simulink model "TestMultirotorSimPx4v1_8"  (R2018b)
settings: Solver=VariableStepAuto  StartTime=0.0  StopTime=Simulation.T_END  MaxStep=Simulation.TS_MAX  RelTol=1e-3  EnableMultiTasking=on
PreLoadFcn:
  | % InitializeParameters;
undefined symbols (not defined in the file): Aero, armed, ctrl_state, Initial, Motor, Simulation, Uav, v_att_sp, v_control_mode
libraries: QuaternionLibrary x13, simulink_extras x9, Px4Library x3, dspsigattribs x1, dspstat3 x1, simulink x1
(part 3 of 9)

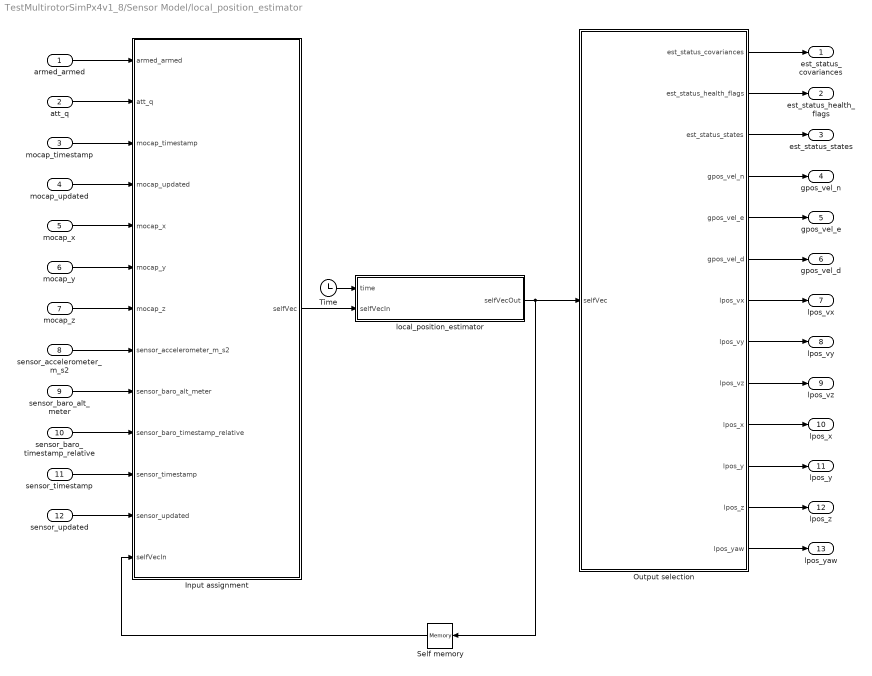
== system TestMultirotorSimPx4v1_8/Sensor Model/local_position_estimator ==
  armed_armed : Inport
  att_q : Inport  Port=2
  mocap_timestamp : Inport  Port=3
  mocap_updated : Inport  Port=4
  mocap_x : Inport  Port=5
  mocap_y : Inport  Port=6
  mocap_z : Inport  Port=7
  sensor_accelerometer_m_s2 : Inport  Port=8
  sensor_baro_alt_meter : Inport  Port=9
  sensor_baro_timestamp_relative : Inport  Port=10
  sensor_timestamp : Inport  Port=11
  sensor_updated : Inport  Port=12
  Input assignment : MATLAB Function  TreatAsAtomicUnit=on
  Output selection : MATLAB Function  TreatAsAtomicUnit=on
  Self memory : Memory  InitialCondition=[0, 0, 0, 0, 0, 0, 0, 0, 0, 0, 0, 0, 0, 0, 0, 0, 0, 0, 0, 0, 0, 0, 0, 0, 0, 0, 0, 0, 0, 0, 0, 0, 0, 0, 0, 0, 0, 0, 0, 0, 0, 0, 0, 0, 0, 0, 0, 0, 0, 0, 0, 0, 0, 0, 0, 0, 0, 0, 0, 0, 0, 0, 0, 0, 0, 0, 0, 0, 0, 0, 0, 0, 0, 0, 0, 0, 0, 0, 0, 0, 0, 0, 0, 0, 0, 0, 0, 0, 0, 0, 0, 0, 0, 0, 0, 0, 0, 0, 0, 0, 0, 0, 0, 0, 0, 0, 0, 0, 0, 0, 0, 0, 0, 0, 0, 0, 0, 0, 0, 0, 0, 0, 0, 0, 0, 0, 0, 0, 0, 0, 0, 8.82050518214, 12.094592431, 13.9876612368, 16.0875642296, 17.8797700658, 19.6465647819, 1e-1, 2.0, 2.0, 2.0, 2^2, 2^0, 2^1, 2^7, 2^1, 2^6, 2^0, 2^4, 2^5, 2^2, 2^3, 0, 10.0, 8, 0, 0, 0, 0, 0, 0, 0, 0, 0, 0, 8, 0, 0, 0, 0, 0, 0, 0, 0, 0, 0, 8, 0, 0, 0, 0, 0, 0, 0, 0, 0, 0, 2*LPE_VXY_PUB*LPE_VXY_PUB, 0, 0, 0, 0, 0, 0, 0, 0, 0, 0, 2*LPE_VXY_PUB*LPE_VXY_PUB, 0, 0, 0, 0, 0, 0, 0, 0, 0, 0, 2*LPE_VXY_PUB*LPE_VXY_PUB, 0, 0, 0, 0, 0, 0, 0, 0, 0, 0, 1e-6, 0, 0, 0, 0, 0, 0, 0, 0, 0, 0, 1e-6, 0, 0, 0, 0, 0, 0, 0, 0, 0, 0, 1e-6, 0, 0, 0, 0, 0, 0, 0, 0, 0, 0, 8, 1.0e6, 0, 0, 0, 0, 0, 0, 0, 0, 0, 0, 0, 0, 0, 0, 0, 0, 0, 0, 0, 0, 0, 0, 0, 0, 0, 0, 0, 0, 0, 0, 0, 0, 0, 0, 0, 0, 0, 0, 0, 0, 0, 0, 0, 0, 0, 0, 0, 0, 0, 0, 0, 0, 0, 0, 0, 0, 0, 0, 0, 0, 0, 0, 0, 0, 0, 0, 0, 0, 0, 0, 0, 0, 0, 0, 0, 0, 0, 0, 0, 0, 0, 0, 0, 0, 0, 0, 0, 0, 0, 0, 0, 0, 0, 0, 0, 0, 0, 0, 0, 0, 0, 0, 0, 0, 0, 0, 0, 0, 0, 0, 0, 0, 0, 0, 0, 0, 0, 0, 2^0, 2^3, 2^1, 2^7, 2^2, 2^6, 2^4, 2^5, 0, LPE_ACC_XY, 0, LPE_ACC_Z, LPE_SAMPLING_PERIOD, LPE_X_LP, 0, 0, 0, 0, 0, 0, LPE_BAR_Z, LPE_SAMPLING_PERIOD, 0, 0, 0, 0, LPE_FAKE_ORIGIN, 0, LPE_FGYRO_HP, LPE_FGYRO_HP, LPE_FLW_QMIN, LPE_FLW_R, LPE_FLW_RR, LPE_FLW_SCALE, LPE_FLW_OFF_Z, LPE_FUSION, 0, LPE_GPS_DELAY, LPE_EPH_MAX, LPE_EPV_MAX, LPE_GPS_VXY, LPE_GPS_VZ, LPE_GPS_XY, LPE_GPS_Z, LPE_LAT, LPE_LON, 0, 0, LPE_LAND_VXY, LPE_LAND_Z, 0, LPE_LDR_OFF_Z, LPE_LDR_Z, 0, 0, 0, 0, 0, 0, 0, LPE_VIC_P, LPE_PN_B, LPE_PN_P, LPE_PN_T, LPE_PN_V, 8, 0, 0, 0, 0, 0, 0, 0, 0, 0, 0, 0, 0, 0, 0, 0, 0, 0, 0, 0, 0, 0, 0, 0, 0, 0, 0, 0, 0, 0, 0, 0, 0, 0, 0, 0, 0, 0, 0, 0, 0, 0, 0, 0, 0, 0, 0, 0, 0, 0, 0, 0, 0, 0, 0, 0, 0, 0, 0, 0, 0, 0, 0, 0, 0, 0, 0, 0, 0, 0, 0, 0, 0, 0, 0, 255, 0, LPE_SNR_OFF_Z, LPE_SNR_Z, 0, 0, 0, 0, 0, 0, 0, 0, 0, 0, 0, 0, 0, 0, 0, 0, 0, 0, 0, 0, 0, 0, 0, 0, 0, 0, 0, 0, 0, 0, 0, 0, 0, 0, 0, 0, 0, 0, 0, 1, 1, LPE_T_MAX_GRADE, 0, 0, 0, 0, 0, 0, 0, 0, 0, 0, 0, LPE_VIS_DELAY, LPE_VIS_XY, LPE_VIS_Z, LPE_VXY_PUB, 0, 0, 0, 0, 0, 0, 0, 0, 0, 0, 0, 0, 0, 0, 0, 0, 0, 0, 0, 0, 0, 0, 0, 0, 0, 0, 0, 0, 0, 0, 0, 0, 0, 0, 0, 0, 0, 0, 0, 0, 0, 0, 0, 0, 0, 0, 0, 0, 0, 0, 0, 0, 0, 0, 0, 0, 0, 0, 0, 0, 0, 0, 0, 0, 0, 0, 0, 0, 0, 0, 0, 0, 0, 0, 0, 0, 0, 0, 0, 0, 0, 0, 0, 0, 0, 0, 0, 0, 0, 0, 0, 0, 0, 0, 0, 0, 0, 0, 0, 0, 0, 0, 0, 0, 0, 0, 0, 0, 0, 0, 1, 1, LPE_SAMPLING_PERIOD, LPE_X_LP, 0, 0, 0, 0, 0, 0, 0, 0, 0, 0, LPE_Z_PUB]
  Time : Clock
  local_position_estimator : MATLAB Function  TreatAsAtomicUnit=on  SystemSampleTime=LPE_SAMPLING_PERIOD
  est_status_covariances : Outport
  est_status_health_flags : Outport  Port=2
  est_status_states : Outport  Port=3
  gpos_vel_n : Outport  Port=4
  gpos_vel_e : Outport  Port=5
  gpos_vel_d : Outport  Port=6
  lpos_vx : Outport  Port=7
  lpos_vy : Outport  Port=8
  lpos_vz : Outport  Port=9
  lpos_x : Outport  Port=10
  lpos_y : Outport  Port=11
  lpos_z : Outport  Port=12
  lpos_yaw : Outport  Port=13
  wires:
  Output selection/13(lpos_yaw) -> lpos_yaw/1
  Output selection/12(lpos_z) -> lpos_z/1
  Output selection/11(lpos_y) -> lpos_y/1
  Output selection/10(lpos_x) -> lpos_x/1
  Output selection/9(lpos_vz) -> lpos_vz/1
  Output selection/8(lpos_vy) -> lpos_vy/1
  Output selection/7(lpos_vx) -> lpos_vx/1
  Output selection/6(gpos_vel_d) -> gpos_vel_d/1
  Output selection/5(gpos_vel_e) -> gpos_vel_e/1
  Output selection/4(gpos_vel_n) -> gpos_vel_n/1
  Output selection/3(est_status_states) -> est_status_states/1
  Output selection/2(est_status_health_flags) -> est_status_health_flags/1
  Output selection/1(est_status_covariances) -> est_status_covariances/1
  sensor_updated/1 -> Input assignment/12(sensor_updated)
  sensor_timestamp/1 -> Input assignment/11(sensor_timestamp)
  sensor_baro_timestamp_relative/1 -> Input assignment/10(sensor_baro_timestamp_relative)
  sensor_baro_alt_meter/1 -> Input assignment/9(sensor_baro_alt_meter)
  sensor_accelerometer_m_s2/1 -> Input assignment/8(sensor_accelerometer_m_s2)
  mocap_z/1 -> Input assignment/7(mocap_z)
  mocap_y/1 -> Input assignment/6(mocap_y)
  mocap_x/1 -> Input assignment/5(mocap_x)
  mocap_updated/1 -> Input assignment/4(mocap_updated)
  mocap_timestamp/1 -> Input assignment/3(mocap_timestamp)
  att_q/1 -> Input assignment/2(att_q)
  armed_armed/1 -> Input assignment/1(armed_armed)
  Time/1 -> local_position_estimator/1(time)
  Self memory/1 -> Input assignment/13(selfVecIn)
  local_position_estimator/1(selfVecOut) -> Self memory/1, Output selection/1(selfVec)
  Input assignment/1(selfVec) -> local_position_estimator/2(selfVecIn)

== system TestMultirotorSimPx4v1_8/att_mixerInput/Euler Angles to Quaternion ==
  euler : Inport
  MATLAB Function : MATLAB Function  TreatAsAtomicUnit=on
  quaternion : Outport
  wires:
  MATLAB Function/1(quat) -> quaternion/1
  euler/1 -> MATLAB Function/1(eulerAngles)

== system TestMultirotorSimPx4v1_8/att_mixerInput/Quaternion to Euler Angles2 ==
  quaternion : Inport
  MATLAB Function : MATLAB Function  TreatAsAtomicUnit=on
  euler : Outport
  wires:
  quaternion/1 -> MATLAB Function/1(quat)
  MATLAB Function/1(eul) -> euler/1

== system TestMultirotorSimPx4v1_8/att_mixerInput/Quaternion to Euler Angles3 ==
  quaternion : Inport
  MATLAB Function : MATLAB Function  TreatAsAtomicUnit=on
  euler : Outport
  wires:
  quaternion/1 -> MATLAB Function/1(quat)
  MATLAB Function/1(eul) -> euler/1

== system TestMultirotorSimPx4v1_8/mc_att_control/Flags ==
  armed : Inport
  control_attitude : Inport  Port=2
  control_auto : Inport  Port=3
  control_manual : Inport  Port=4
  control_rates : Inport  Port=5
  control_velocity : Inport  Port=6
  BusIn : Inport  Port=7
  Flags bus assignment : BusAssignment  AssignedSignals=armed.armed,v_control_mode.flag_control_attitude_enabled,v_control_mode.flag_control_auto_enabled,v_control_mode.flag_control_manual_enabled,v_control_mode.flag_control_rates_enabled,v_control_mode.flag_control_velocity_enabled
  Bus : Outport
  wires:
  control_rates/1 -> Flags bus assignment/6
  control_manual/1 -> Flags bus assignment/5
  control_attitude/1 -> Flags bus assignment/3
  armed/1 -> Flags bus assignment/2
  control_velocity/1 -> Flags bus assignment/7
  control_auto/1 -> Flags bus assignment/4
  BusIn/1 -> Flags bus assignment/1
  Flags bus assignment/1 -> Bus/1

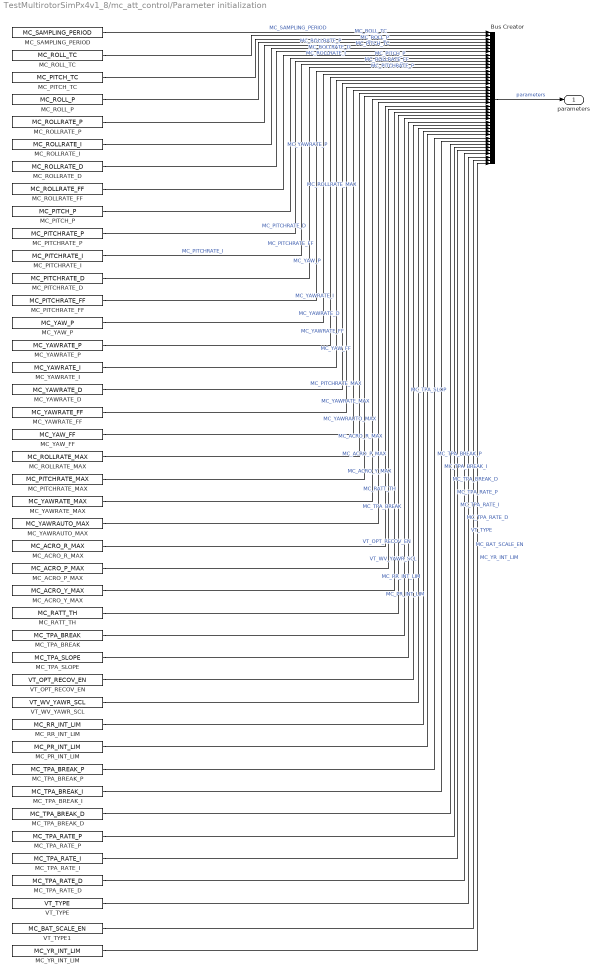
== system TestMultirotorSimPx4v1_8/mc_att_control/Parameter initialization ==
  Bus Creator : BusCreator  Inputs='MC_SAMPLING_PERIOD','MC_ROLL_TC','MC_PITCH_TC','MC_ROLL_P','MC_ROLLRATE_P','MC_ROLLRATE_I','MC_ROLLRATE_D','MC_ROLLRATE_FF','MC_PITCH_P','MC_PITCHRATE_P','MC_PITCHRATE_I','MC_PITCHRATE_D','MC_PITCHRATE_FF','MC_YAW_P','MC_YAWRATE_P','MC_YAWRATE_I','MC_YAWRATE_D','MC_YAWRATE_FF','MC_YAW_FF','MC_ROLLRATE_MAX','MC_PITCHRATE_MAX','MC_YAWRATE_MAX','MC_YAWRAUTO_MAX','MC_ACRO_R_MAX','MC_ACRO_P_MAX','MC_ACRO_Y_MAX','MC_RATT_TH','MC_TPA_BREAK','MC_TPA_SLOP','VT_OPT_RECOV_EN','VT_WV_YAWR_SCL','MC_RR_INT_LIM','MC_PR_INT_LIM','MC_TPA_BREAK_P','MC_TPA_BREAK_I','MC_TPA_BREAK_D','MC_TPA_RATE_P','MC_TPA_RATE_I','MC_TPA_RATE_D','VT_TYPE','MC_BAT_SCALE_EN','MC_YR_INT_LIM'  OutDataTypeStr=Bus: parameterBus
  MC_ACRO_P_MAX : Constant  Value=MC_ACRO_P_MAX
  MC_ACRO_R_MAX : Constant  Value=MC_ACRO_R_MAX
  MC_ACRO_Y_MAX : Constant  Value=MC_ACRO_Y_MAX
  MC_PITCHRATE_D : Constant  Value=MC_PITCHRATE_D
  MC_PITCHRATE_FF : Constant  Value=MC_PITCHRATE_FF
  MC_PITCHRATE_I : Constant  Value=MC_PITCHRATE_I
  MC_PITCHRATE_MAX : Constant  Value=MC_PITCHRATE_MAX
  MC_PITCHRATE_P : Constant  Value=MC_PITCHRATE_P
  MC_PITCH_P : Constant  Value=MC_PITCH_P
  MC_PITCH_TC : Constant  Value=MC_PITCH_TC
  MC_PR_INT_LIM : Constant  Value=MC_PR_INT_LIM
  MC_RATT_TH : Constant  Value=MC_RATT_TH
  MC_ROLLRATE_D : Constant  Value=MC_ROLLRATE_D
  MC_ROLLRATE_FF : Constant  Value=MC_ROLLRATE_FF
  MC_ROLLRATE_I : Constant  Value=MC_ROLLRATE_I
  MC_ROLLRATE_MAX : Constant  Value=MC_ROLLRATE_MAX
  MC_ROLLRATE_P : Constant  Value=MC_ROLLRATE_P
  MC_ROLL_P : Constant  Value=MC_ROLL_P
  MC_ROLL_TC : Constant  Value=MC_ROLL_TC
  MC_RR_INT_LIM : Constant  Value=MC_RR_INT_LIM
  MC_SAMPLING_PERIOD : Constant  Value=MC_SAMPLING_PERIOD
  MC_TPA_BREAK : Constant  Value=MC_TPA_BREAK
  MC_TPA_BREAK_D : Constant  Value=MC_TPA_BREAK_D
  MC_TPA_BREAK_I : Constant  Value=MC_TPA_BREAK_I
  MC_TPA_BREAK_P : Constant  Value=MC_TPA_BREAK_P
  MC_TPA_RATE_D : Constant  Value=MC_TPA_RATE_D
  MC_TPA_RATE_I : Constant  Value=MC_TPA_RATE_I
  MC_TPA_RATE_P : Constant  Value=MC_TPA_RATE_P
  MC_TPA_SLOPE : Constant  Value=MC_TPA_SLOPE
  MC_YAWRATE_D : Constant  Value=MC_YAWRATE_D
  MC_YAWRATE_FF : Constant  Value=MC_YAWRATE_FF
  MC_YAWRATE_I : Constant  Value=MC_YAWRATE_I
  MC_YAWRATE_MAX : Constant  Value=MC_YAWRATE_MAX
  MC_YAWRATE_P : Constant  Value=MC_YAWRATE_P
  MC_YAWRAUTO_MAX : Constant  Value=MC_YAWRAUTO_MAX
  MC_YAW_FF : Constant  Value=MC_YAW_FF
  MC_YAW_P : Constant  Value=MC_YAW_P
  MC_YR_INT_LIM : Constant  Value=MC_YR_INT_LIM
  VT_OPT_RECOV_EN : Constant  Value=VT_OPT_RECOV_EN
  VT_TYPE : Constant  Value=VT_TYPE
  VT_TYPE1 : Constant  Value=MC_BAT_SCALE_EN
  VT_WV_YAWR_SCL : Constant  Value=VT_WV_YAWR_SCL
  parameters : Outport
  wires:
  MC_RR_INT_LIM/1 -> Bus Creator/32  "MC_RR_INT_LIM"
  VT_TYPE1/1 -> Bus Creator/41  "MC_BAT_SCALE_EN"
  MC_TPA_BREAK_D/1 -> Bus Creator/36  "MC_TPA_BREAK_D"
  MC_TPA_BREAK_I/1 -> Bus Creator/35  "MC_TPA_BREAK_I"
  MC_TPA_BREAK_P/1 -> Bus Creator/34  "MC_TPA_BREAK_P"
  MC_YR_INT_LIM/1 -> Bus Creator/42  "MC_YR_INT_LIM"
  MC_TPA_RATE_D/1 -> Bus Creator/39  "MC_TPA_RATE_D"
  VT_TYPE/1 -> Bus Creator/40  "VT_TYPE"
  MC_TPA_BREAK/1 -> Bus Creator/28  "MC_TPA_BREAK"
  VT_WV_YAWR_SCL/1 -> Bus Creator/31  "VT_WV_YAWR_SCL"
  MC_TPA_SLOPE/1 -> Bus Creator/29  "MC_TPA_SLOP"
  MC_ACRO_R_MAX/1 -> Bus Creator/24  "MC_ACRO_R_MAX"
  Bus Creator/1 -> parameters/1  "parameters"
  MC_ACRO_P_MAX/1 -> Bus Creator/25  "MC_ACRO_P_MAX"
  MC_ACRO_Y_MAX/1 -> Bus Creator/26  "MC_ACRO_Y_MAX"
  VT_OPT_RECOV_EN/1 -> Bus Creator/30  "VT_OPT_RECOV_EN"
  MC_RATT_TH/1 -> Bus Creator/27  "MC_RATT_TH"
  MC_YAWRATE_MAX/1 -> Bus Creator/22  "MC_YAWRATE_MAX"
  MC_YAWRAUTO_MAX/1 -> Bus Creator/23  "MC_YAWRAUTO_MAX"
  MC_YAWRATE_P/1 -> Bus Creator/15  "MC_YAWRATE_P"
  MC_ROLL_TC/1 -> Bus Creator/2  "MC_ROLL_TC"
  MC_PITCH_P/1 -> Bus Creator/9  "MC_PITCH_P"
  MC_PITCH_TC/1 -> Bus Creator/3  "MC_PITCH_TC"
  MC_SAMPLING_PERIOD/1 -> Bus Creator/1  "MC_SAMPLING_PERIOD"
  MC_PITCHRATE_MAX/1 -> Bus Creator/21  "MC_PITCHRATE_MAX"
  MC_YAWRATE_I/1 -> Bus Creator/16  "MC_YAWRATE_I"
  MC_ROLL_P/1 -> Bus Creator/4  "MC_ROLL_P"
  MC_ROLLRATE_MAX/1 -> Bus Creator/20  "MC_ROLLRATE_MAX"
  MC_YAW_P/1 -> Bus Creator/14  "MC_YAW_P"
  MC_YAWRATE_FF/1 -> Bus Creator/18  "MC_YAWRATE_FF"
  MC_ROLLRATE_FF/1 -> Bus Creator/8  "MC_ROLLRATE_FF"
  MC_PITCHRATE_D/1 -> Bus Creator/12  "MC_PITCHRATE_D"
  MC_PITCHRATE_I/1 -> Bus Creator/11  "MC_PITCHRATE_I"
  MC_ROLLRATE_D/1 -> Bus Creator/7  "MC_ROLLRATE_D"
  MC_ROLLRATE_P/1 -> Bus Creator/5  "MC_ROLLRATE_P"
  MC_PITCHRATE_P/1 -> Bus Creator/10  "MC_PITCHRATE_P"
  MC_PITCHRATE_FF/1 -> Bus Creator/13  "MC_PITCHRATE_FF"
  MC_YAW_FF/1 -> Bus Creator/19  "MC_YAW_FF"
  MC_YAWRATE_D/1 -> Bus Creator/17  "MC_YAWRATE_D"
  MC_ROLLRATE_I/1 -> Bus Creator/6  "MC_ROLLRATE_I"
  MC_PR_INT_LIM/1 -> Bus Creator/33  "MC_PR_INT_LIM"
  MC_TPA_RATE_P/1 -> Bus Creator/37  "MC_TPA_RATE_P"
  MC_TPA_RATE_I/1 -> Bus Creator/38  "MC_TPA_RATE_I"

== system TestMultirotorSimPx4v1_8/Sensor Model/Accelerometer1/Quaternion to Rotation Matrix ==
  quaternion : Inport
  MATLAB Function : MATLAB Function  TreatAsAtomicUnit=on
  rotationMatrix : Outport
  wires:
  MATLAB Function/1(R) -> rotationMatrix/1
  quaternion/1 -> MATLAB Function/1(q)

== matlab function TestMultirotorSimPx4v1_8/Quadrotor Quaternion Model/Equations of motion ==
  data: VBody input; VBodyDot output; nuBody input; Q input; TBody input size=3; tauBody input size=3; F_D input size=3; M_D input size=3; time input; nuBodyDot output; Uav parameter; xiDDot output; Simulation parameter
function [VBodyDot, nuBodyDot, xiDDot] = QuadrotorQuaternionModel(...
    VBody, nuBody, Q, TBody, tauBody, F_D, M_D, time, Uav, Simulation)
%#codegen

%% Handle 2D pitch test
if isfield( Uav, 'PITCH_ONLY') && Uav.PITCH_ONLY
    tauBody = [0; 1; 0] .* tauBody;
    M_D = [0; 1; 0] .* M_D;
end

if isfield( Simulation, 'T_START_STEP') && ( time < Simulation.T_START_STEP )
    tauBody = [0; 0; 0] .* tauBody;
    M_D = [0; 0; 0] .* M_D;
end

%% Moments and Forces
% Body frame accelerations
VBodyDot  = (1/Uav.M) * (Q'*Uav.G + TBody - cross(nuBody, Uav.M*VBody) + F_D);
nuBodyDot = Uav.I \ (tauBody - cross(nuBody, Uav.I*nuBody) + M_D);

% Inertial frame accelerations
xiDDot = (1/Uav.M)*(Uav.G + Q*(TBody + F_D));
% etaDDot = WInvertDot*nuBody + WInvert*nuBodyDot;

% Check centripetal force in inertial frame
% F_C = R*cross(nuBody,m*VBody);

if Uav.PITCH_ONLY
    xiDDot = [1; 1; 0] .* xiDDot;
end

end

== matlab function TestMultirotorSimPx4v1_8/Compute Sph ==
  data: V_appBody input; azimuth output; elevation output; radius output
function [azimuth, elevation, radius] = computeSph(V_appBody)
%#codegen

% Convert from polar to spherical coordinates
[ azimuth, elevation, radius ] = cart2sph( V_appBody(1), V_appBody(2), V_appBody(3) );

== matlab function TestMultirotorSimPx4v1_8/att_controller_ff ==
  data: Textra input; thrustDes output [0..1]; V_appBody input size=3; q input; omega input; Motor parameter; Uav parameter; Aero parameter
function thrustDes  = ffThrust( Textra, V_appBody, q, omega, Motor, Uav, Aero )
%#codegen
    [ azimuth, elevation, windSpeed ] = cart2sph( V_appBody(1), V_appBody(2), V_appBody(3) );
    
    R = QuatToRot(q);
    Rz = R(:,3);
    vertical = [0; 0; 1];
    
    alpha = atan2( norm(cross( Rz, vertical )), dot( Rz, vertical ) );

    if strcmp( Aero.Type, 'Body oriented' )
        U = windSpeed;
        lambda = mean(omega .* Uav.D_PROP / ( 2 * U ));
        
        Cz1 = dot( Aero.Cz1.coefs, [sin(alpha), 1] );
        fz_lift = 0.5 .* Uav.RHO_AIR .* U^2 .* Cz1 * Uav.A_UAV;

        Cz2 = dot( Aero.Cz2.coefs, [alpha, 1]);
        p = Aero.Cz3.coefs;
        Cz3 = p(1) * sin(alpha) + p(2) * ( 1 - exp(-p(3).*lambda) ) .* sin(3*alpha) + ...
            p(4);
        a = 0.5 .* Uav.RHO_AIR .* Cz2 .* Uav.D_PROP^2 .* Uav.A_PROP; % Rotor thrust
        b = 0.5 .* Uav.RHO_AIR .* Cz3 .* U .* Uav.D_PROP .* Uav.A_PROP; % Rotor thrust correction
        
        mg = Uav.G(3);
        Trequired = ((mg / cos(alpha)) - (fz_lift) + Textra)/Uav.N_ROTORS;
        c = Trequired;
        
        omegaRefDes = (-b + sqrt(b^2 + 4*a*c) )/(2*a);
    else
        % Thrust
        x1 = sin(-elevation);
        x2 = windSpeed;
        CT1 = 0.5 * Uav.RHO_AIR * dot( Aero.CT1.coefs, [ 1, x1, x2, x1*x2, x1^2, x2^2, x1^2*x2^2  ] );
        CT2 = 0.5 * Uav.RHO_AIR * dot( Aero.CT2.coefs, [ 1, x1, x2, x1*x2, x1^2, x2^2, x1^2*x2^2  ] );

        % Drag
        x1 = cos(-elevation);
        x2 = mean(omega);
        Cd1 = dot( Aero.Cd1.coefs, [ 1, x1, x2, x1*x2, x1^2, x2^2, x1^2*x2^2  ] );
        Cd2 = dot( Aero.Cd2.coefs, [ 1, x1, x2, x1*x2, x1^2, x2^2, x1^2*x2^2  ] );
        f_D = 0.5 * Uav.RHO_AIR * Cd1 * windSpeed^2 + ...
        0.5 * Uav.RHO_AIR * Cd2 * windSpeed;

        % Lift
        x1 = -elevation;
        x2 = 0;
        Cl = dot( Aero.Cl.coefs, [ 1, x1, x2, x1*x2, x1^2, x2^2, x1^2*x2^2  ] );
        f_l = 0.5 * Uav.RHO_AIR * Cl * windSpeed^2;

        F_D = zeros(3,1);
        F_l = zeros(3,1);
        [ F_D(1), F_D(2), F_D(3) ] = sph2cart( azimuth, elevation, f_D );
        [ F_l(1), F_l(2), F_l(3) ] = sph2cart( azimuth, elevation + pi/2, f_l );

        mg = -Uav.G(3);
        Trequired = mg / cos(alpha) - (F_l(3) + F_D(3)) + Textra;

        omegaRefDes = (-CT2 + sqrt(CT2^2 + 4*CT1*Trequired) )/(2*CT1);
    end


    omegaDes = omegaRefDes; %- mean(omegaDot)*7.006512e-02;
    pwmDes = ( omegaDes/0.84 + 6.528579e2) / 7.969173e-1;

    thrustDes = (pwmDes - 1000) / 1000;
end

function R = QuatToRot( q )
% QUATERNIONTOROTATIONMATRIXMAT Convert quaternion to rotation matrix
% Written by: J.X.J. Bannwarth, 27/03/17
    W = q(1);
    X = q(2);
    Y = q(3);
    Z = q(4);
    
    xx = X * X;
    xy = X * Y;
    xz = X * Z;
    xw = X * W;

    yy = Y * Y;
    yz = Y * Z;
    yw = Y * W;
    
    zz = Z * Z;
    zw = Z * W;

    m00 = 1 - 2 * ( yy + zz );
    m01 =     2 * ( xy - zw );
    m02 =     2 * ( xz + yw );

    m10 =     2 * ( xy + zw );
    m11 = 1 - 2 * ( xx + zz );
    m12 =     2 * ( yz - xw );

    m20 =     2 * ( xz - yw );
    m21 =     2 * ( yz + xw );
    m22 = 1 - 2 * ( xx + yy );
    
    R = [m00 m01 m02;
         m10 m11 m12;
         m20 m21 m22];
    
end

== matlab function TestMultirotorSimPx4v1_8/Applied wind speed/Relative velocity ==
  data: nuBody input; Uav parameter; VMotorRelBody output
function VMotorRelBody = relativeMotorVelocity( nuBody , Uav )
%#codegen
    VMotorRelBody = cross( nuBody, Uav.L_VEC );
end

== matlab function TestMultirotorSimPx4v1_8/Applied wind speed/Compute V_app2 ==
  data: Q input; UBody output; U input size=3
function UBody = computeUBody(Q, U)
%#codegen

% Rotation matrix from Wind frame to Inertial frame
% Wind frame SEU, inertial frame NED
R_U = [1,  0, 0;
       0, -1, 0;
       0,  0, 1];
   
UBody = Q' * R_U * U;

== matlab function TestMultirotorSimPx4v1_8/att_mixerInput/Euler Angles to Quaternion/MATLAB Function ==
  data: eulerAngles input; quat output
function quat   = EulerToQuaternion( eulerAngles )
%EULERTOQUATERNION Convert Euler angles to a quaternion
%   Based on PX4 Firmware code: https://github.com/PX4/Firmware
%   Written by: J.X.J. Bannwarth
%   Last modified: 29/08/2016

    roll  = eulerAngles(1);
    pitch = eulerAngles(2);
    yaw   = eulerAngles(3);

    cosPhi_2   = cos(roll / 2.0);
    sinPhi_2   = sin(roll / 2.0);
    cosTheta_2 = cos(pitch / 2.0);
    sinTheta_2 = sin(pitch / 2.0);
    cosPsi_2   = cos(yaw / 2.0);
    sinPsi_2   = sin(yaw / 2.0);

    quat = [ cosPhi_2 .* cosTheta_2 .* cosPsi_2 + sinPhi_2 .* sinTheta_2 .* sinPsi_2;
             sinPhi_2 .* cosTheta_2 .* cosPsi_2 - cosPhi_2 .* sinTheta_2 .* sinPsi_2;
             cosPhi_2 .* sinTheta_2 .* cosPsi_2 + sinPhi_2 .* cosTheta_2 .* sinPsi_2;
             cosPhi_2 .* cosTheta_2 .* sinPsi_2 - sinPhi_2 .* sinTheta_2 .* cosPsi_2 ];

end

== matlab function TestMultirotorSimPx4v1_8/Sensor Model/Global reprojection/map_projection_reproject ==
  data: x input; y input; lat output; lon output; LAT0 parameter; LON0 parameter
function [ lat, lon ] = map_projection_reproject( x, y, LAT0, LON0)
%#codegen
%MAP_PROJECTION_REPROJECT
    M_DEG_TO_RAD = 0.017453292519943295;
	ref.lat_rad = LAT0 * M_DEG_TO_RAD;
	ref.lon_rad = LON0 * M_DEG_TO_RAD;
	ref.sin_lat = 0;
	ref.cos_lat = 0; 
    ref.sin_lat = sin(ref.lat_rad);
    ref.cos_lat = cos(ref.lat_rad);
    
    CONSTANTS_RADIUS_OF_EARTH = 6371000;
    M_PI = 3.14159265358979323846;

    x_rad = x / CONSTANTS_RADIUS_OF_EARTH;
    y_rad = y / CONSTANTS_RADIUS_OF_EARTH;
    c = sqrt(x_rad * x_rad + y_rad * y_rad);
    
    sin_c = sin(c);
    cos_c = cos(c);

    if (abs(c) > eps)
        lat_rad = asin(cos_c * ref.sin_lat + (x_rad * sin_c * ref.cos_lat) / c);
        lon_rad = (ref.lon_rad + atan2(y_rad * sin_c, c * ref.cos_lat * cos_c - x_rad * ref.sin_lat * sin_c));
    else
        lat_rad = ref.lat_rad;
        lon_rad = ref.lon_rad;
    end

    lat = lat_rad * 180.0 / M_PI;
    lon = lon_rad * 180.0 / M_PI;
end

== matlab function TestMultirotorSimPx4v1_8/att_mixerInput/Quaternion to Euler Angles3/MATLAB Function ==
  data: quat input; eul output
function eul   = QuaternionToEuler( quat )
%QUATERNIONTOEULER Convert quaternion to euler angles
%   Based on PX4 Firmware code: https://github.com/PX4/Firmware
%   Written by:    J.X.J. Bannwarth, 2016/08/29
%   Last modified: J.X.J. Bannwarth, 2018/12/11

    eul = [ atan2(2.0 .* (quat(1) .* quat(2) + quat(3) .* quat(4)), ...
                1.0 - 2.0 .* (quat(2) .* quat(2) + quat(3) .* quat(3)));
	        asin(2.0 .* (quat(1) .* quat(3) - quat(4) .* quat(2)));
            atan2(2.0 .* (quat(1) .* quat(4) + quat(2) .* quat(3)), ...
                1.0 - 2.0 .* (quat(3) .* quat(3) + quat(4) .* quat(4))) ];
end

== matlab function TestMultirotorSimPx4v1_8/Sensor Model/attitude_estimator_q/Input assignment q ==
  data: airspeed_sub_indicated_airspeed_m_s input; airspeed_sub_timestamp input; global_pos_sub_eph input; global_pos_sub_lat input; global_pos_sub_lon input; global_pos_sub_timestamp input; global_pos_sub_vel_n input; global_pos_sub_vel_e input; global_pos_sub_vel_d input; mocap_sub_q input; mocap_sub_timestamp input; sensors_sub_timestamp input; sensors_sub_gyro_rad input; sensors_sub_accelerometer_m_s2 input; sensors_sub_accelerometer_timestamp_relative input; sensors_sub_magnetometer_ga input; sensors_sub_magnetometer_timestamp_relative input; selfVecIn input; selfVec output
function selfVec = InputAssignment( ...
	     airspeed_sub_indicated_airspeed_m_s, ...
	                  airspeed_sub_timestamp, ...
	                      global_pos_sub_eph, ...
	                      global_pos_sub_lat, ...
	                      global_pos_sub_lon, ...
	                global_pos_sub_timestamp, ...
	                    global_pos_sub_vel_n, ...
	                    global_pos_sub_vel_e, ...
	                    global_pos_sub_vel_d, ...
	                             mocap_sub_q, ...
	                     mocap_sub_timestamp, ...
	                   sensors_sub_timestamp, ...
	                    sensors_sub_gyro_rad, ...
	          sensors_sub_accelerometer_m_s2, ...
	sensors_sub_accelerometer_timestamp_relative, ...
	             sensors_sub_magnetometer_ga, ...
	sensors_sub_magnetometer_timestamp_relative, ...
	                               selfVecIn ...
	)
%#codegen

	selfVec = selfVecIn;

	% Variable assignment
	selfVec(10:10) =      airspeed_sub_indicated_airspeed_m_s;
	selfVec(11:11) =                   airspeed_sub_timestamp;
	selfVec(45:45) =                       global_pos_sub_eph;
	selfVec(46:46) =                       global_pos_sub_lat;
	selfVec(47:47) =                       global_pos_sub_lon;
	selfVec(48:48) =                 global_pos_sub_timestamp;
	selfVec(50:50) =                     global_pos_sub_vel_n;
	selfVec(51:51) =                     global_pos_sub_vel_e;
	selfVec(52:52) =                     global_pos_sub_vel_d;
	selfVec(147:150) =                              mocap_sub_q;
	selfVec(151:151) =                      mocap_sub_timestamp;
	selfVec(166:166) =                    sensors_sub_timestamp;
	selfVec(168:170) =                     sensors_sub_gyro_rad;
	selfVec(171:173) =           sensors_sub_accelerometer_m_s2;
	selfVec(174:174) = sensors_sub_accelerometer_timestamp_relative;
	selfVec(175:177) =              sensors_sub_magnetometer_ga;
	selfVec(178:178) = sensors_sub_magnetometer_timestamp_relative;
end

== matlab function TestMultirotorSimPx4v1_8/Sensor Model/attitude_estimator_q/Output selection q ==
  data: att_pub_timestamp output; att_pub_rollspeed output; att_pub_pitchspeed output; att_pub_yawspeed output; att_pub_q output; selfVec input; ctrl_state_pub_x_acc output; ctrl_state_pub_y_acc output; ctrl_state_pub_z_acc output
function [ ...
                        att_pub_timestamp, ...
                        att_pub_rollspeed, ...
                       att_pub_pitchspeed, ...
                         att_pub_yawspeed, ...
                                att_pub_q, ...
                     ctrl_state_pub_x_acc, ...
                     ctrl_state_pub_y_acc, ...
                     ctrl_state_pub_z_acc] ...
   = OutputSelection( selfVec )
%#codegen

	% Variable assignment
	                       att_pub_timestamp = selfVec(14:14);
	                       att_pub_rollspeed = selfVec(15:15);
	                      att_pub_pitchspeed = selfVec(16:16);
	                        att_pub_yawspeed = selfVec(17:17);
	                               att_pub_q = selfVec(18:21);
	                    ctrl_state_pub_x_acc = selfVec(29:29);
	                    ctrl_state_pub_y_acc = selfVec(30:30);
	                    ctrl_state_pub_z_acc = selfVec(31:31);
end
